simulink model "MAIN_SIMULINK_2023a"  (R2024b)
settings: Solver=ode45  StartTime=0.0  StopTime=800  RelTol=1e-7  EnableMultiTasking=on
values from neighbouring files (symbols this model uses):
  f = 1/5    (= 0.2)    [Copy_of_auto_identification.m]    (also in not_done_identification.m)
  gp_1 = gp_1/Gain_tec    [Copy_of_auto_identification.m]    (also in not_done_identification.m = gp_1 / Gain_tec)
undefined symbols (not defined in the file or in its folder): DFz, gp_2, gp_3, gpp_t1, gpp_t2, gpp_t3, kc, Tiz, truc, Z_T1T3, Z_T3
libraries: simulink_extras x5, simulink x1
settings Model: Creator=LiberT  LastModifiedBy=lordo
settings SolverCC: AlgebraicLoopSolver=TrustRegion
settings DataIOCC: LimitDataPoints=on  SaveFormat=Array  SignalLoggingSaveFormat=ModelDataLogs  ReturnWorkspaceOutputs=off
settings OptimizationCC: BlockReduction=off  BooleanDataType=off  ExpressionDepthLimit=2147483647  InitFltsAndDblsToZero=on  LifeSpan=inf
settings DebuggingCC: SaveWithParameterizedLinksMsg=none  UnderspecifiedInitializationDetection=Classic  MergeDetectMultiDrivingBlocksExec=none  SignalResolutionControl=TryResolveAllWithWarning  MultiTaskDSMMsg=warning  MultiTaskCondExecSysMsg=none  FcnCallInpInsideContextMsg=warning  UnconnectedInputMsg=warning  UnconnectedOutputMsg=warning  UnconnectedLineMsg=warning  StateNameClashWarn=warning  SFUnexpectedBacktrackingDiag=warning  SFNoUnconditionalDefaultTransitionDiag=warning  SFExecutionAtInitializationDiag=none  ArithmeticOperatorsInVariantConditions=warning
settings HardwareCC: ProdBitPerPointer=32  ProdBitPerSizeT=32  ProdBitPerPtrDiffT=32  ProdLargestAtomicFloat=None  ProdIntDivRoundTo=Undefined  ProdEndianess=Unspecified  ProdWordSize=32  ProdHWDeviceType=32-bit Generic  TargetUnknown=on
settings ModelReferenceCC: EnableRefExpFcnMdlSchedulingChecks=on  PropagateSignalLabelsOutOfModel=off
settings SFSimCC: SimUseLocalCustomCode=off  LegacyBehaviorForPersistentVarInContinuousTime=on  CustomCodeUndefinedFunction=UseInterfaceOnly
settings RTWCC: RTWUseLocalCustomCode=off  GPUComputeCapability=3.5
settings CodeAppCC: StateflowObjectComments=on
settings GRTTargetCC: TargetFcnLib=ansi_tfl_tmw.mat  TargetLangStandard=C89/C90 (ANSI)  ModelReferenceCompliant=off  CompOptLevelCompliant=off  CombineOutputUpdateFcns=off  MatFileLogging=off  GRTInterface=on
settings ConfigComp: CovMetricSettings=dw  CovSaveCumulativeToWorkspaceVar=on  CovSaveSingleToWorkspaceVar=on  CovExternalEMLEnable=off

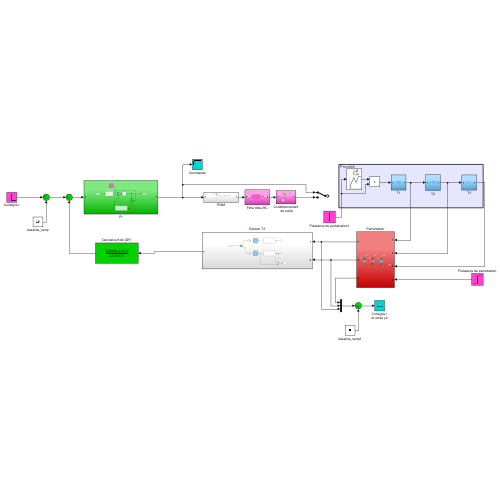
[thumbnail: Simulink's stored preview of the top-level diagram]
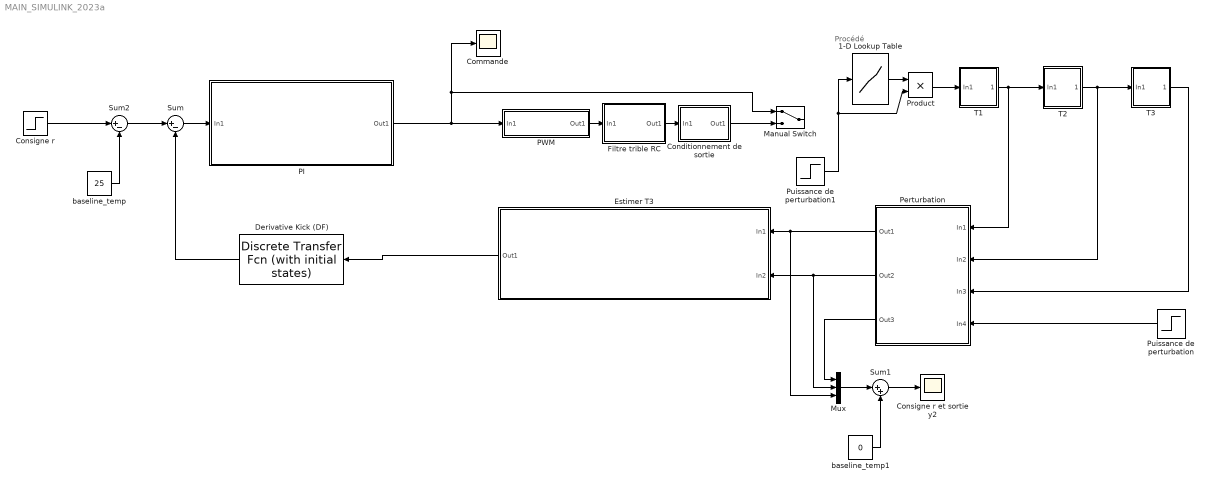
== system MAIN_SIMULINK_2023a ==
  note: Procédé
  1-D Lookup Table : Lookup_n-D  NumberOfTableDimensions=1  BreakpointsForDimension1=[-0.8, -0.6, -0.4, -0.2, 0.1, 0.2, 0.4, 0.6, 0.8]  Table=[1.12, 1.62, 1.865, 2.15, 1.72, 1.72, 2.22, 2.22, 2.22]  InternalRulePriority=Speed  RndMeth=Simplest
  Commande : Scope
  Conditionnement de sortie : Subsystem
  Consigne r : Step  Time=700  Before=30  After=20  SampleTime=0
  Consigne r et sortie y2 : Scope
  Derivative Kick (DF) : simulink_extras/Additional Discrete/Discrete Transfer Fcn (with initial states)  N=DFz.num{1}  D=DFz.den{1}  X0=[0]  TS=1/f
  Estimer T3 : Subsystem
  Filtre trible RC : Subsystem
  Manual Switch : ManualSwitch
  Mux : Mux  Inputs=3
  PI : Subsystem
  PWM : Subsystem
  Perturbation : Subsystem
  Product : Product
  Puissance de perturbation : Step  Time=500  After=0  SampleTime=0
  Puissance de perturbation1 : Step  Time=0  Before=truc{1}  After=truc{1}  SampleTime=0
  Sum : Sum  Inputs=|+-  InputSameDT=on  SaturateOnIntegerOverflow=on  OutDataTypeStr=Inherit: Same as first input
  Sum1 : Sum  Inputs=|++  InputSameDT=on  SaturateOnIntegerOverflow=on  OutDataTypeStr=Inherit: Same as first input
  Sum2 : Sum  Inputs=|+-  InputSameDT=on  SaturateOnIntegerOverflow=on  OutDataTypeStr=Inherit: Same as first input
  T1 : Subsystem
  T2 : Subsystem
  T3 : Subsystem
  baseline_temp : Constant  Value=25
  baseline_temp1 : Constant  Value=0
  wires:
  Consigne r/1 -> Sum2/1
  baseline_temp/1 -> Sum2/2
  Sum2/1 -> Sum/1
  PI/1(Out1) -> Manual Switch/1, Commande/1, PWM/1(In1)
  Sum/1 -> PI/1(In1)
  PWM/1(Out1) -> Filtre trible RC/1(In1)
  Filtre trible RC/1(Out1) -> Conditionnement de sortie/1(In1)
  Conditionnement de sortie/1(Out1) -> Manual Switch/2
  Derivative Kick (DF)/1 -> Sum/2
  T2/1(Out1) -> Perturbation/2(In2), T3/1(In1)
  T1/1(Out1) -> Perturbation/1(In1), T2/1(In1)
  Estimer T3/1(Out1) -> Derivative Kick (DF)/1
  T3/1(Out1) -> Perturbation/3(In3)
  Puissance de perturbation/1 -> Perturbation/4(In4)
  Perturbation/1(Out1) -> Mux/3, Estimer T3/1(In1)
  Perturbation/2(Out2) -> Mux/2, Estimer T3/2(In2)
  Perturbation/3(Out3) -> Mux/1
  1-D Lookup Table/1 -> Product/1
  Puissance de perturbation1/1 -> Product/2, 1-D Lookup Table/1
  Product/1 -> T1/1(In1)
  Mux/1 -> Sum1/1
  baseline_temp1/1 -> Sum1/2
  Sum1/1 -> Consigne r et sortie y2/1

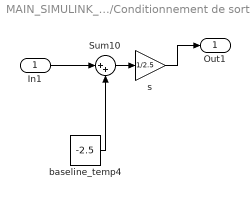
== system MAIN_SIMULINK_2023a/Conditionnement de sortie ==
  In1 : Inport
  Sum10 : Sum  Inputs=|++  InputSameDT=on  SaturateOnIntegerOverflow=on  OutDataTypeStr=Inherit: Same as first input
  baseline_temp4 : Constant  Value=-2.5
  s : Gain  Gain=1/2.5
  Out1 : Outport
  wires:
  Sum10/1 -> s/1
  s/1 -> Out1/1
  baseline_temp4/1 -> Sum10/2
  In1/1 -> Sum10/1

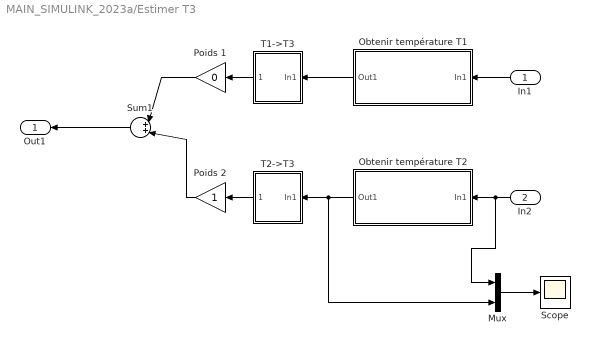
== system MAIN_SIMULINK_2023a/Estimer T3 ==
  In1 : Inport
  In2 : Inport  Port=2
  Mux : Mux  Inputs=2
  Obtenir température T1 : Subsystem
  Obtenir température T2 : Subsystem
  Poids 1 : Gain  Gain=0
  Poids 2 : Gain
  Scope : Scope
  Sum1 : Sum  Inputs=|++|  InputSameDT=on  SaturateOnIntegerOverflow=on  OutDataTypeStr=Inherit: Same as first input
  T1->T3 : Subsystem
  T2->T3 : Subsystem
  Out1 : Outport
  wires:
  Poids 2/1 -> Sum1/2
  Obtenir température T2/1(Out1) -> Mux/2, T2->T3/1(In1)
  T1->T3/1(Out1) -> Poids 1/1
  T2->T3/1(Out1) -> Poids 2/1
  In1/1 -> Obtenir température T1/1(In1)
  Obtenir température T1/1(Out1) -> T1->T3/1(In1)
  Poids 1/1 -> Sum1/1
  Sum1/1 -> Out1/1
  In2/1 -> Mux/1, Obtenir température T2/1(In1)
  Mux/1 -> Scope/1

== system MAIN_SIMULINK_2023a/Filtre trible RC ==
  In1 : Inport
  Filtre triple RC : TransferFcn  Denominator=[ (4e-3)^3, 5*(4e-3)^2, 6*4e-3, 1]
  Out1 : Outport
  wires:
  Filtre triple RC/1 -> Out1/1
  In1/1 -> Filtre triple RC/1

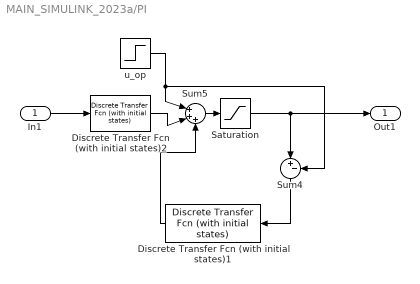
== system MAIN_SIMULINK_2023a/PI ==
  In1 : Inport
  Discrete Transfer Fcn (with initial states)1 : simulink_extras/Additional Discrete/Discrete Transfer Fcn (with initial states)  N=Tiz.num{1}  D=Tiz.den{1}  X0=[0]  TS=1/f
  Discrete Transfer Fcn (with initial states)2 : simulink_extras/Additional Discrete/Discrete Transfer Fcn (with initial states)  N=kc  D=1  X0=[0]  TS=1/f
  Saturation : Saturate  UpperLimit=1  LowerLimit=-1
  Sum4 : Sum  Inputs=|+-  InputSameDT=on  SaturateOnIntegerOverflow=on  OutDataTypeStr=Inherit: Same as first input
  Sum5 : Sum  Inputs=|+++  InputSameDT=on  SaturateOnIntegerOverflow=on  OutDataTypeStr=Inherit: Same as first input
  u_op : Step  Time=0  After=0  SampleTime=0
  Out1 : Outport
  wires:
  u_op/1 -> Sum5/1, Sum4/2
  Discrete Transfer Fcn (with initial states)1/1 -> Sum5/3
  Saturation/1 -> Out1/1, Sum4/1
  Sum5/1 -> Saturation/1
  In1/1 -> Discrete Transfer Fcn (with initial states)2/1
  Discrete Transfer Fcn (with initial states)2/1 -> Sum5/2
  Sum4/1 -> Discrete Transfer Fcn (with initial states)1/1

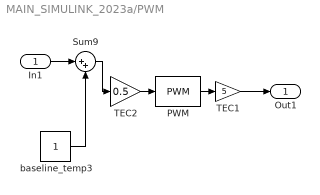
== system MAIN_SIMULINK_2023a/PWM ==
  In1 : Inport
  PWM : simulink/Discontinuities/PWM  DisableCoverage=on  Period=1  InitialDelay=0  DisallowZeroDutyCycle=off  RunAtFixedTimeIntervals=off  SampleTime=0.1
  Sum9 : Sum  Inputs=|++  InputSameDT=on  SaturateOnIntegerOverflow=on  OutDataTypeStr=Inherit: Same as first input
  TEC1 : Gain  Gain=5
  TEC2 : Gain  Gain=0.5
  baseline_temp3 : Constant
  Out1 : Outport
  wires:
  TEC1/1 -> Out1/1
  PWM/1 -> TEC1/1
  TEC2/1 -> PWM/1
  Sum9/1 -> TEC2/1
  baseline_temp3/1 -> Sum9/2
  In1/1 -> Sum9/1

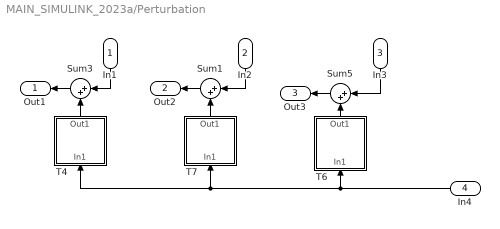
== system MAIN_SIMULINK_2023a/Perturbation ==
  In1 : Inport
  In2 : Inport  Port=2
  In3 : Inport  Port=3
  In4 : Inport  Port=4
  Sum1 : Sum  Inputs=|++  InputSameDT=on  SaturateOnIntegerOverflow=on  OutDataTypeStr=Inherit: Same as first input
  Sum3 : Sum  Inputs=|++  InputSameDT=on  SaturateOnIntegerOverflow=on  OutDataTypeStr=Inherit: Same as first input
  Sum5 : Sum  Inputs=|++  InputSameDT=on  SaturateOnIntegerOverflow=on  OutDataTypeStr=Inherit: Same as first input
  T4 : Subsystem
  T6 : Subsystem
  T7 : Subsystem
  Out1 : Outport
  Out2 : Outport  Port=2
  Out3 : Outport  Port=3
  wires:
  In4/1 -> T6/1(In1), T7/1(In1), T4/1(In1)
  Sum1/1 -> Out2/1
  T6/1(Out1) -> Sum5/2
  T7/1(Out1) -> Sum1/2
  Sum5/1 -> Out3/1
  In2/1 -> Sum1/1
  T4/1(Out1) -> Sum3/2
  Sum3/1 -> Out1/1
  In3/1 -> Sum5/1
  In1/1 -> Sum3/1

== system MAIN_SIMULINK_2023a/T1 ==
  In1 : Inport
  Dynamique1 : TransferFcn  Numerator=gp_1.num{1}  Denominator=gp_1.den{1}
  Out1 : Outport
  wires:
  In1/1 -> Dynamique1/1
  Dynamique1/1 -> Out1/1

== system MAIN_SIMULINK_2023a/T2 ==
  In1 : Inport
  Dynamique1 : TransferFcn  Numerator=gp_2.num{1}  Denominator=gp_2.den{1}
  Retard2 : TransportDelay  DelayTime=gp_2.IODelay  BufferSize=20000
  Out1 : Outport
  wires:
  Dynamique1/1 -> Out1/1
  In1/1 -> Retard2/1
  Retard2/1 -> Dynamique1/1

== system MAIN_SIMULINK_2023a/T3 ==
  In1 : Inport
  Dynamique3 : TransferFcn  Numerator=gp_3.Numerator{1}  Denominator=gp_3.Denominator{1}
  Retard3 : TransportDelay  DelayTime=gp_3.IODelay  BufferSize=20000
  Out1 : Outport
  wires:
  Dynamique3/1 -> Out1/1
  Retard3/1 -> Dynamique3/1
  In1/1 -> Retard3/1

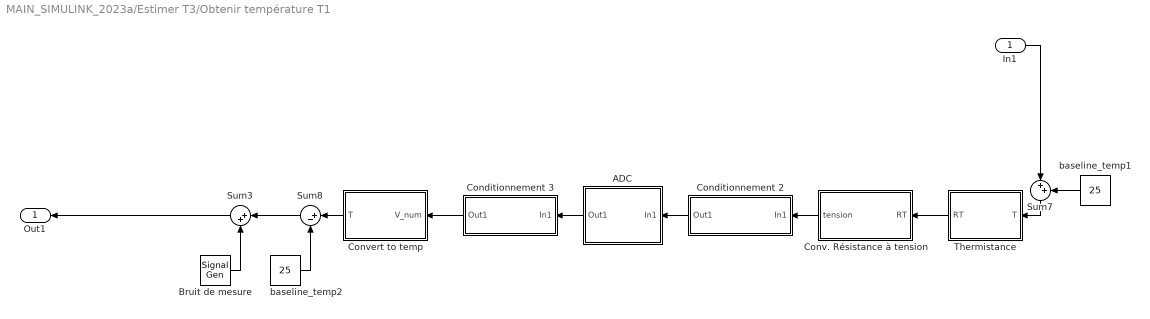
== system MAIN_SIMULINK_2023a/Estimer T3/Obtenir température T1 ==
  In1 : Inport
  ADC : Subsystem
  Bruit de mesure : SignalGenerator  Amplitude=0  Units=rad/sec
  Conditionnement 2 : Subsystem
  Conditionnement 3 : Subsystem
  Conv. Résistance à tension : MATLAB Function  TreatAsAtomicUnit=on
  Convert to temp : MATLAB Function  TreatAsAtomicUnit=on
  Sum3 : Sum  Inputs=|++  InputSameDT=on  SaturateOnIntegerOverflow=on  OutDataTypeStr=Inherit: Same as first input
  Sum7 : Sum  Inputs=|++  InputSameDT=on  SaturateOnIntegerOverflow=on  OutDataTypeStr=Inherit: Same as first input
  Sum8 : Sum  Inputs=|+-  InputSameDT=on  SaturateOnIntegerOverflow=on  OutDataTypeStr=Inherit: Same as first input
  Thermistance : MATLAB Function  TreatAsAtomicUnit=on
  baseline_temp1 : Constant  Value=25
  baseline_temp2 : Constant  Value=25
  Out1 : Outport
  wires:
  baseline_temp2/1 -> Sum8/2
  ADC/1(Out1) -> Conditionnement 3/1(In1)
  Thermistance/1(RT) -> Conv. Résistance à tension/1(RT)
  Conditionnement 2/1(Out1) -> ADC/1(In1)
  Conv. Résistance à tension/1(tension) -> Conditionnement 2/1(In1)
  Sum7/1 -> Thermistance/1(T)
  Conditionnement 3/1(Out1) -> Convert to temp/1(V_num)
  Convert to temp/1(T) -> Sum8/1
  baseline_temp1/1 -> Sum7/2
  Bruit de mesure/1 -> Sum3/2
  In1/1 -> Sum7/1
  Sum3/1 -> Out1/1
  Sum8/1 -> Sum3/1

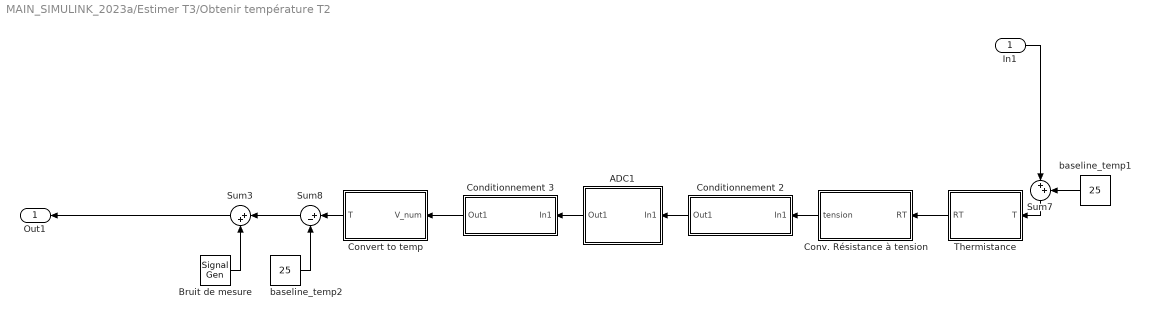
== system MAIN_SIMULINK_2023a/Estimer T3/Obtenir température T2 ==
  In1 : Inport
  ADC1 : Subsystem
  Bruit de mesure : SignalGenerator  Amplitude=0  Units=rad/sec
  Conditionnement 2 : Subsystem
  Conditionnement 3 : Subsystem
  Conv. Résistance à tension : MATLAB Function  TreatAsAtomicUnit=on
  Convert to temp : MATLAB Function  TreatAsAtomicUnit=on
  Sum3 : Sum  Inputs=|++  InputSameDT=on  SaturateOnIntegerOverflow=on  OutDataTypeStr=Inherit: Same as first input
  Sum7 : Sum  Inputs=|++  InputSameDT=on  SaturateOnIntegerOverflow=on  OutDataTypeStr=Inherit: Same as first input
  Sum8 : Sum  Inputs=|+-  InputSameDT=on  SaturateOnIntegerOverflow=on  OutDataTypeStr=Inherit: Same as first input
  Thermistance : MATLAB Function  TreatAsAtomicUnit=on
  baseline_temp1 : Constant  Value=25
  baseline_temp2 : Constant  Value=25
  Out1 : Outport
  wires:
  baseline_temp2/1 -> Sum8/2
  Sum8/1 -> Sum3/1
  ADC1/1(Out1) -> Conditionnement 3/1(In1)
  Thermistance/1(RT) -> Conv. Résistance à tension/1(RT)
  Conditionnement 2/1(Out1) -> ADC1/1(In1)
  Conv. Résistance à tension/1(tension) -> Conditionnement 2/1(In1)
  Sum7/1 -> Thermistance/1(T)
  Conditionnement 3/1(Out1) -> Convert to temp/1(V_num)
  Convert to temp/1(T) -> Sum8/1
  baseline_temp1/1 -> Sum7/2
  Bruit de mesure/1 -> Sum3/2
  In1/1 -> Sum7/1
  Sum3/1 -> Out1/1

== system MAIN_SIMULINK_2023a/Estimer T3/T1->T3 ==
  In1 : Inport
  Delay : Delay  DelayLength=Z_T1T3.IODelay  InitialCondition=0
  t3_t2 : simulink_extras/Additional Discrete/Discrete Transfer Fcn (with initial states)  N=Z_T1T3.num{1}  D=Z_T1T3.den{1}  X0=[0]  TS=1/f
  Out1 : Outport
  wires:
  t3_t2/1 -> Out1/1
  In1/1 -> Delay/1
  Delay/1 -> t3_t2/1

== system MAIN_SIMULINK_2023a/Estimer T3/T2->T3 ==
  In1 : Inport
  Delay : Delay  DelayLength=Z_T3.IODelay  InitialCondition=0
  Derivative Kick (DF) : simulink_extras/Additional Discrete/Discrete Transfer Fcn (with initial states)  N=Z_T3.num{1}  D=Z_T3.den{1}  X0=[0]  TS=1/f
  Out1 : Outport
  wires:
  In1/1 -> Delay/1
  Delay/1 -> Derivative Kick (DF)/1
  Derivative Kick (DF)/1 -> Out1/1

== system MAIN_SIMULINK_2023a/Perturbation/T4 ==
  In1 : Inport
  Dynamique1 : TransferFcn  Numerator=gpp_t1.num{1}  Denominator=gpp_t1.den{1}
  Out1 : Outport
  wires:
  Dynamique1/1 -> Out1/1
  In1/1 -> Dynamique1/1

== system MAIN_SIMULINK_2023a/Perturbation/T6 ==
  In1 : Inport
  Dynamique1 : TransferFcn  Numerator=gpp_t3.num{1}  Denominator=gpp_t3.den{1}
  Retard2 : TransportDelay  DelayTime=gpp_t3.IODelay  BufferSize=5000
  Out1 : Outport
  wires:
  Dynamique1/1 -> Retard2/1
  Retard2/1 -> Out1/1
  In1/1 -> Dynamique1/1

== system MAIN_SIMULINK_2023a/Perturbation/T7 ==
  In1 : Inport
  Dynamique1 : TransferFcn  Numerator=gpp_t2.num{1}  Denominator=gpp_t2.den{1}
  Out1 : Outport
  wires:
  In1/1 -> Dynamique1/1
  Dynamique1/1 -> Out1/1

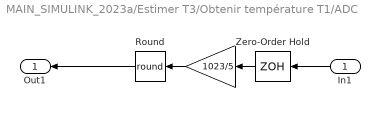
== system MAIN_SIMULINK_2023a/Estimer T3/Obtenir température T1/ADC ==
  In1 : Inport
  " " : Gain  Gain=1023/5
  Round : Rounding  Operator=round
  Zero-Order Hold : ZeroOrderHold  SampleTime=-1
  Out1 : Outport
  wires:
  " "/1 -> Round/1
  Zero-Order Hold/1 -> " "/1
  In1/1 -> Zero-Order Hold/1
  Round/1 -> Out1/1

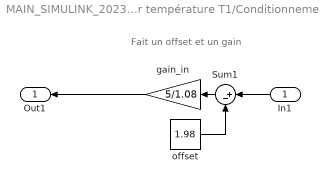
== system MAIN_SIMULINK_2023a/Estimer T3/Obtenir température T1/Conditionnement 2 ==
  note: Fait un offset et un gain
  In1 : Inport
  Sum1 : Sum  Inputs=|+-  InputSameDT=on  SaturateOnIntegerOverflow=on  OutDataTypeStr=Inherit: Same as first input
  gain_in : Gain  Gain=5/1.08
  offset : Constant  Value=1.98
  Out1 : Outport
  wires:
  gain_in/1 -> Out1/1
  offset/1 -> Sum1/2
  Sum1/1 -> gain_in/1
  In1/1 -> Sum1/1

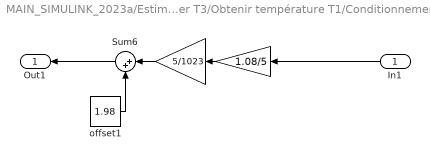
== system MAIN_SIMULINK_2023a/Estimer T3/Obtenir température T1/Conditionnement 3 ==
  In1 : Inport
  "  " : Gain  Gain=1.08/5
  "   " : Gain  Gain=5/1023
  Sum6 : Sum  Inputs=|++  InputSameDT=on  SaturateOnIntegerOverflow=on  OutDataTypeStr=Inherit: Same as first input
  offset1 : Constant  Value=1.98
  Out1 : Outport
  wires:
  "  "/1 -> "   "/1
  offset1/1 -> Sum6/2
  "   "/1 -> Sum6/1
  Sum6/1 -> Out1/1
  In1/1 -> "  "/1

== system MAIN_SIMULINK_2023a/Estimer T3/Obtenir température T2/ADC1 ==
  In1 : Inport
  " " : Gain  Gain=1023/5
  Round : Rounding  Operator=round
  Zero-Order Hold : ZeroOrderHold  SampleTime=-1
  Out1 : Outport
  wires:
  " "/1 -> Round/1
  Zero-Order Hold/1 -> " "/1
  In1/1 -> Zero-Order Hold/1
  Round/1 -> Out1/1

== system MAIN_SIMULINK_2023a/Estimer T3/Obtenir température T2/Conditionnement 2 ==
  note: Fait un offset et un gain
  In1 : Inport
  Sum1 : Sum  Inputs=|+-  InputSameDT=on  SaturateOnIntegerOverflow=on  OutDataTypeStr=Inherit: Same as first input
  gain_in : Gain  Gain=5/1.08
  offset : Constant  Value=1.98
  Out1 : Outport
  wires:
  gain_in/1 -> Out1/1
  offset/1 -> Sum1/2
  Sum1/1 -> gain_in/1
  In1/1 -> Sum1/1

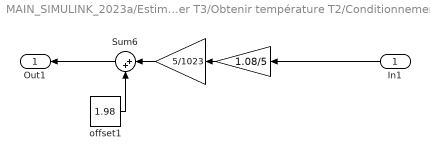
== system MAIN_SIMULINK_2023a/Estimer T3/Obtenir température T2/Conditionnement 3 ==
  In1 : Inport
  "  " : Gain  Gain=1.08/5
  "   " : Gain  Gain=5/1023
  Sum6 : Sum  Inputs=|++  InputSameDT=on  SaturateOnIntegerOverflow=on  OutDataTypeStr=Inherit: Same as first input
  offset1 : Constant  Value=1.98
  Out1 : Outport
  wires:
  "  "/1 -> "   "/1
  offset1/1 -> Sum6/2
  "   "/1 -> Sum6/1
  Sum6/1 -> Out1/1
  In1/1 -> "  "/1

== matlab function MAIN_SIMULINK_2023a/Estimer T3/Obtenir température T1/Convert to temp ==
  data: V_num input; T output
function T = v2t(V_num)
% Définition des coefficients
Rfixe = 10000;
RT = Rfixe / (5.0 /V_num - 1.0);
R25 = 10000;
lnR = log(RT / R25);   
A = 0.00335401643468053;
B = 0.000256523550896126;
C = 0.00000260597012072052;
D = 0.000000063292612648746;


T = (1.0 / (A + B * lnR + C * lnR * lnR + D * lnR * lnR * lnR)) - 273.15;
end

== matlab function MAIN_SIMULINK_2023a/Estimer T3/Obtenir température T1/Thermistance ==
  data: T input; RT output
function RT = t2r(T)
% Définition des coefficients

A = -14.65719769;
B = 4798.84200000;
C = -115334.00000000;
D = -3730535.00000000;
R25 = 10000; % Exemple de R25 (à adapter selon ton besoin)


% Calcul de la résistance
RT = R25 * exp(A + B/(T+273.15) + C/(T+273.15)^2 + D/(T+273.15)^3);
end

== matlab function MAIN_SIMULINK_2023a/Estimer T3/Obtenir température T2/Conv. Résistance à tension ==
  data: RT input; tension output
function tension = r2v(RT)
% Définition des coefficients
Rfixe = 10000;
tension = 5*(RT)/(RT+Rfixe);
end

== matlab function MAIN_SIMULINK_2023a/Estimer T3/Obtenir température T2/Convert to temp ==
  data: V_num input; T output
function T = v2t(V_num)
% Définition des coefficients
Rfixe = 10000;
RT = Rfixe / (5.0 /V_num - 1.0);
R25 = 10000;
lnR = log(RT / R25);   
A = 0.00335401643468053;
B = 0.000256523550896126;
C = 0.00000260597012072052;
D = 0.000000063292612648746;
T = (1.0 / (A + B * lnR + C * lnR * lnR + D * lnR * lnR * lnR)) - 273.15;
end

== matlab function MAIN_SIMULINK_2023a/Estimer T3/Obtenir température T2/Thermistance ==
  data: T input; RT output
function RT = t2r(T)
% Définition des coefficients
A = -14.65719769;
B = 4798.84200000;
C = -115334.00000000;
D = -3730535.00000000;
R25 = 10000; % Exemple de R25 (à adapter selon ton besoin)

% Calcul de la résistance
RT = R25 * exp(A + B/(T+273.15) + C/(T+273.15)^2 + D/(T+273.15)^3);
end

== matlab function MAIN_SIMULINK_2023a/Estimer T3/Obtenir température T1/Conv. Résistance à tension ==
  data: RT input; tension output
function tension = r2v(RT)
% Définition des coefficients
Rfixe = 10000;
tension = 5*(RT)/(RT+Rfixe);
end
